simulink model "aero_guidance_airframe"  (R2018a)
settings: Solver=ode45  StartTime=0.0  StopTime=10.0  RelTol=1e-3  AbsTol=1e-6
PreLoadFcn:
  | aero_guid_dat
undefined symbols (not defined in the file): alpha_vec, Cm_alpha, Cm_el, Cm_q, Cx_alpha, Cz_alpha, Cz_el, d_ref, g, h_ini, Mach_vec, S_ref, Thrust, x_ini
libraries: aerospace x3
Description:
  | Vehicle Airframe + Atmosphere Model
settings Model: ExtModeTrigMode=oneshot  ExtModeArmWhenConnect=off  ExtModeAutoUpdateStatusClock=off  Creator=The MathWorks, Inc.  LastModifiedBy=The MathWorks, Inc.
settings SolverCC: AutoScaleAbsTol=off
settings DataIOCC: SaveFormat=Array  SignalLoggingName=logsOut
settings OptimizationCC: BlockReduction=off  BooleanDataType=off  ExpressionDepthLimit=2147483647  InitFltsAndDblsToZero=on  LifeSpan=inf
settings DebuggingCC: SaveWithParameterizedLinksMsg=none  CheckExecutionContextPreStartOutputMsg=on  CheckExecutionContextRuntimeOutputMsg=on  SignalResolutionControl=TryResolveAllWithWarning  MultiTaskDSMMsg=warning  MultiTaskCondExecSysMsg=none  FcnCallInpInsideContextMsg=warning  StateNameClashWarn=warning  SFUnexpectedBacktrackingDiag=warning  SFNoUnconditionalDefaultTransitionDiag=warning  SFExecutionAtInitializationDiag=none
settings HardwareCC: ProdBitPerPointer=32  ProdBitPerSizeT=32  ProdBitPerPtrDiffT=32  ProdLargestAtomicFloat=None  ProdIntDivRoundTo=Undefined  ProdEndianess=Unspecified  ProdWordSize=32  ProdHWDeviceType=32-bit Generic
settings ModelReferenceCC: UpdateModelReferenceTargets=IfOutOfDate  PropagateSignalLabelsOutOfModel=off
settings CodeAppCC: StateflowObjectComments=on
settings GRTTargetCC: TargetFcnLib=ansi_tfl_tmw.mat  TargetLangStandard=C89/C90 (ANSI)  GeneratePreprocessorConditionals=Disable all  CombineOutputUpdateFcns=off  GRTInterface=on
settings ConfigComp: CovMetricSettings=dw  CovHtmlReporting=on  CovSaveCumulativeToWorkspaceVar=on  CovSaveSingleToWorkspaceVar=on  CovExternalEMLEnable=off

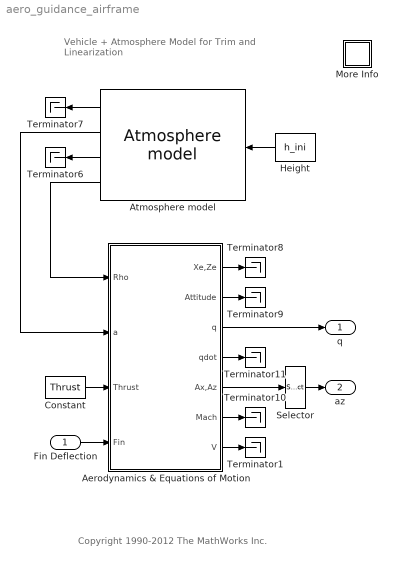
== system aero_guidance_airframe ==
  note: Vehicle + Atmosphere Model
      | for Trim and Linearization
  note: Copyright 1990-2012 The MathWorks Inc.
  Fin Deflection : Inport
  Aerodynamics & Equations of Motion : Subsystem
  Atmosphere model : aerospace/Atmosphere/Atmosphere model
      settings: SourceProductName=Simulink  SourceProductBaseCode=SL
  Constant : Constant  Value=Thrust
  Height : Constant  Value=h_ini
  More Info : Subsystem
      settings: OpenFcn=showdemo('aero_guidance_trimlinearize')
      mask Display: disp('?')
  Selector : Selector  InputPortWidth=2  IndexOptions=Index vector (dialog)  Indices=[2]  OutputSizes=1
  Terminator{1,6..11} (7 alike) : Terminator
  q : Outport  InitialOutput=0
  az : Outport  Port=2  InitialOutput=0
  wires:
  Height/1 -> Atmosphere model/1
  Atmosphere model/1 -> Terminator7/1
  Atmosphere model/3 -> Terminator6/1
  Constant/1 -> Aerodynamics & Equations of Motion/3(Thrust)
  Fin Deflection/1 -> Aerodynamics & Equations of Motion/4(Fin)
  Aerodynamics & Equations of Motion/1(Xe,Ze) -> Terminator8/1
  Aerodynamics & Equations of Motion/2(Attitude) -> Terminator9/1
  Aerodynamics & Equations of Motion/3(q) -> q/1
  Aerodynamics & Equations of Motion/4(qdot) -> Terminator11/1
  Aerodynamics & Equations of Motion/5(Ax,Az) -> Selector/1
  Aerodynamics & Equations of Motion/6(Mach) -> Terminator10/1
  Aerodynamics & Equations of Motion/7(V) -> Terminator1/1
  Atmosphere model/4 -> Aerodynamics & Equations of Motion/1(Rho)
  Atmosphere model/2 -> Aerodynamics & Equations of Motion/2(a)
  Selector/1 -> az/1

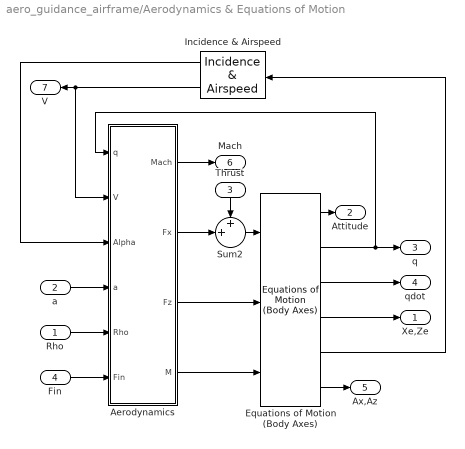
== system aero_guidance_airframe/Aerodynamics & Equations of Motion ==
  Rho : Inport
  a : Inport  Port=2
  Thrust : Inport  Port=3
  Fin : Inport  Port=4
  " Equations of Motion (Body Axes)" : aerospace/3DoF Equations of Motion / Equations of Motion (Body Axes)  v_ini=v_ini  theta_ini=theta_ini  alpha_ini=alpha_ini  q_ini=q_ini  pos_ini=[x_ini -h_ini]  mass=mass  Iyy=Iyy  g=g
      settings: SourceProductName=Simulink  SourceProductBaseCode=SL
  Aerodynamics : Subsystem
  Incidence & Airspeed : aerospace/3DoF Equations of Motion /Incidence  & Airspeed
      settings: SourceProductName=Simulink  SourceProductBaseCode=SL
  Sum2 : Sum  Inputs=++|  SaturateOnIntegerOverflow=on  InputSameDT=on  OutDataTypeStr=Inherit: Same as first input
  Xe,Ze : Outport  InitialOutput=0
  Attitude : Outport  Port=2  InitialOutput=0
  q : Outport  Port=3  InitialOutput=0
  qdot : Outport  Port=4  InitialOutput=0
  Ax,Az : Outport  Port=5  InitialOutput=0
  Mach : Outport  Port=6  InitialOutput=0
  V : Outport  Port=7  InitialOutput=0
  wires:
  " Equations of Motion (Body Axes)"/5 -> Incidence & Airspeed/1
  " Equations of Motion (Body Axes)"/6 -> Ax,Az/1
  " Equations of Motion (Body Axes)"/4 -> Xe,Ze/1
  " Equations of Motion (Body Axes)"/1 -> Attitude/1
  " Equations of Motion (Body Axes)"/3 -> qdot/1
  " Equations of Motion (Body Axes)"/2 -> Aerodynamics/1(q), q/1
  Thrust/1 -> Sum2/1
  Aerodynamics/2(Fx) -> Sum2/2
  Aerodynamics/3(Fz) -> " Equations of Motion (Body Axes)"/2
  Incidence & Airspeed/2 -> Aerodynamics/2(V), V/1
  Fin/1 -> Aerodynamics/6(Fin)
  a/1 -> Aerodynamics/4(a)
  Rho/1 -> Aerodynamics/5(Rho)
  Incidence & Airspeed/1 -> Aerodynamics/3(Alpha)
  Sum2/1 -> " Equations of Motion (Body Axes)"/1
  Aerodynamics/4(" M") -> " Equations of Motion (Body Axes)"/3
  Aerodynamics/1(" Mach") -> Mach/1

== system aero_guidance_airframe/More Info ==

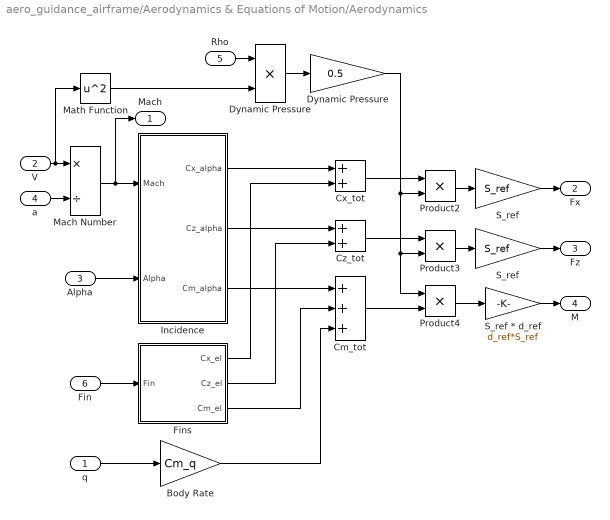
== system aero_guidance_airframe/Aerodynamics & Equations of Motion/Aerodynamics ==
  q : Inport
  V : Inport  Port=2
  Alpha : Inport  Port=3
  a : Inport  Port=4
  Rho : Inport  Port=5
  Fin : Inport  Port=6
  Body Rate : Gain  Gain=Cm_q  SaturateOnIntegerOverflow=on  OutDataTypeStr=Inherit: Same as input  ParamDataTypeStr=Inherit: Same as input
  Cm_tot : Sum  Inputs=+++  SaturateOnIntegerOverflow=on  InputSameDT=on  OutDataTypeStr=Inherit: Same as first input
  Cx_tot : Sum  SaturateOnIntegerOverflow=on  InputSameDT=on  OutDataTypeStr=Inherit: Same as first input
  Cz_tot : Sum  SaturateOnIntegerOverflow=on  InputSameDT=on  OutDataTypeStr=Inherit: Same as first input
  "Dynamic Pressure " : Gain  Gain=0.5  SaturateOnIntegerOverflow=on  OutDataTypeStr=Inherit: Same as input  ParamDataTypeStr=Inherit: Same as input
  Dynamic Pressure : Product  SaturateOnIntegerOverflow=on  RndMeth=Zero  InputSameDT=on  OutDataTypeStr=Inherit: Same as first input
  Fins : Subsystem
  Incidence : Subsystem
  Mach Number : Product  Inputs=*/  SaturateOnIntegerOverflow=on  RndMeth=Zero  InputSameDT=on  OutDataTypeStr=Inherit: Same as first input
  Math Function : Math  Operator=square  SaturateOnIntegerOverflow=on
  Product2 : Product  SaturateOnIntegerOverflow=on  RndMeth=Zero  InputSameDT=on  OutDataTypeStr=Inherit: Same as first input
  Product3 : Product  SaturateOnIntegerOverflow=on  RndMeth=Zero  InputSameDT=on  OutDataTypeStr=Inherit: Same as first input
  Product4 : Product  SaturateOnIntegerOverflow=on  RndMeth=Zero  InputSameDT=on  OutDataTypeStr=Inherit: Same as first input
  S_ref : Gain  Gain=S_ref  SaturateOnIntegerOverflow=on  OutDataTypeStr=Inherit: Same as input  ParamDataTypeStr=Inherit: Same as input
  S_ref * d_ref : Gain  Gain=d_ref*S_ref  SaturateOnIntegerOverflow=on  OutDataTypeStr=Inherit: Same as input  ParamDataTypeStr=Inherit: Same as input
  "S_ref " : Gain  Gain=S_ref  SaturateOnIntegerOverflow=on  OutDataTypeStr=Inherit: Same as input  ParamDataTypeStr=Inherit: Same as input
  " Mach" : Outport  InitialOutput=0
  Fx : Outport  Port=2  InitialOutput=[0]
  Fz : Outport  Port=3  InitialOutput=0
  " M" : Outport  Port=4  InitialOutput=0
  wires:
  Mach Number/1 -> " Mach"/1, Incidence/1(Mach)
  q/1 -> Body Rate/1
  Cm_tot/1 -> Product4/2
  Product4/1 -> S_ref * d_ref/1
  S_ref * d_ref/1 -> " M"/1
  Fin/1 -> Fins/1(Fin)
  "S_ref "/1 -> Fz/1
  Product3/1 -> "S_ref "/1
  S_ref/1 -> Fx/1
  Product2/1 -> S_ref/1
  Cz_tot/1 -> Product3/1
  Cx_tot/1 -> Product2/1
  Alpha/1 -> Incidence/2(Alpha)
  a/1 -> Mach Number/2
  Body Rate/1 -> Cm_tot/3
  Fins/3(Cm_el) -> Cm_tot/2
  Incidence/3(Cm_alpha) -> Cm_tot/1
  Fins/2(Cz_el) -> Cz_tot/2
  Incidence/2(Cz_alpha) -> Cz_tot/1
  Fins/1(Cx_el) -> Cx_tot/2
  Incidence/1(Cx_alpha) -> Cx_tot/1
  V/1 -> Mach Number/1, Math Function/1
  "Dynamic Pressure "/1 -> Product4/1, Product3/2, Product2/2
  Dynamic Pressure/1 -> "Dynamic Pressure "/1
  Rho/1 -> Dynamic Pressure/1
  Math Function/1 -> Dynamic Pressure/2

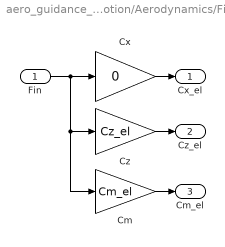
== system aero_guidance_airframe/Aerodynamics & Equations of Motion/Aerodynamics/Fins ==
  Fin : Inport
  Cm : Gain  Gain=Cm_el  SaturateOnIntegerOverflow=on  OutDataTypeStr=Inherit: Same as input  ParamDataTypeStr=Inherit: Same as input
  Cx : Gain  Gain=0  SaturateOnIntegerOverflow=on  OutDataTypeStr=Inherit: Same as input  ParamDataTypeStr=Inherit: Same as input
  Cz : Gain  Gain=Cz_el  SaturateOnIntegerOverflow=on  OutDataTypeStr=Inherit: Same as input  ParamDataTypeStr=Inherit: Same as input
  Cx_el : Outport  InitialOutput=0
  Cz_el : Outport  Port=2  InitialOutput=0
  Cm_el : Outport  Port=3  InitialOutput=0
  wires:
  Cz/1 -> Cz_el/1
  Cm/1 -> Cm_el/1
  Cx/1 -> Cx_el/1
  Fin/1 -> Cz/1, Cm/1, Cx/1

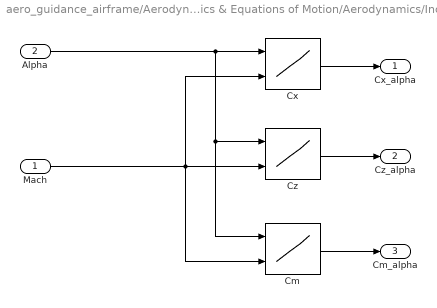
== system aero_guidance_airframe/Aerodynamics & Equations of Motion/Aerodynamics/Incidence ==
  Mach : Inport
  Alpha : Inport  Port=2
  Cm : Lookup_n-D  BreakpointsForDimension1=alpha_vec  BreakpointsForDimension2=Mach_vec  BeginIndexSearchUsingPreviousIndexResult=on  Table=Cm_alpha  InternalRulePriority=Speed  RndMeth=Simplest  InputSameDT=on
  Cx : Lookup_n-D  BreakpointsForDimension1=alpha_vec  BreakpointsForDimension2=Mach_vec  BeginIndexSearchUsingPreviousIndexResult=on  Table=Cx_alpha  InternalRulePriority=Speed  RndMeth=Simplest  InputSameDT=on
  Cz : Lookup_n-D  BreakpointsForDimension1=alpha_vec  BreakpointsForDimension2=Mach_vec  BeginIndexSearchUsingPreviousIndexResult=on  Table=Cz_alpha  InternalRulePriority=Speed  RndMeth=Simplest  InputSameDT=on
  Cx_alpha : Outport  InitialOutput=0
  Cz_alpha : Outport  Port=2  InitialOutput=0
  Cm_alpha : Outport  Port=3  InitialOutput=0
  wires:
  Cx/1 -> Cx_alpha/1
  Cz/1 -> Cz_alpha/1
  Cm/1 -> Cm_alpha/1
  Alpha/1 -> Cx/1, Cm/1, Cz/1
  Mach/1 -> Cx/2, Cm/2, Cz/2
